simulink model "Q2_Model"  (R2016b)
settings: Solver=VariableStepAuto  StartTime=0.0  StopTime=100  RelTol=1e-10  AbsTol=1e-10
values from neighbouring files (symbols this model uses):
  c_a = 0.1    [CSD_HW_1_Script.m]
  D_v = 1e-2    (= 0.01)    [CSD_HW_1_Script.m]
  ddx_height = 5    [CSD_HW_1_Script.m]
  ddx_width = 30/ddx_height    (= 6)    [CSD_HW_1_Script.m]
  gear = 2    [CSD_HW_1_Script.m]
  J = 0.07    [CSD_HW_1_Script.m]
  K_t = 0.46    [CSD_HW_1_Script.m]
  l = 0.3    [CSD_HW_1_Script.m]
  m = 0.8    [CSD_HW_1_Script.m]
  N = 3    [CSD_HW_1_Script.m]    (also in Plotshit.m)
  R = 0.1    [CSD_HW_1_Script.m]    (also in Plotshit.m)
  Step_Height = 0    [CSD_HW_1_Script.m]
  T_sl = 2    [CSD_HW_1_Script.m]
  T_st = 2.6    [CSD_HW_1_Script.m]
  V_max = 20    [CSD_HW_1_Script.m]
undefined symbols (not defined in the file or in its folder): magnitude
libraries: cstblocks x1
settings Model: Creator=nadav  LastModifiedBy=nadav

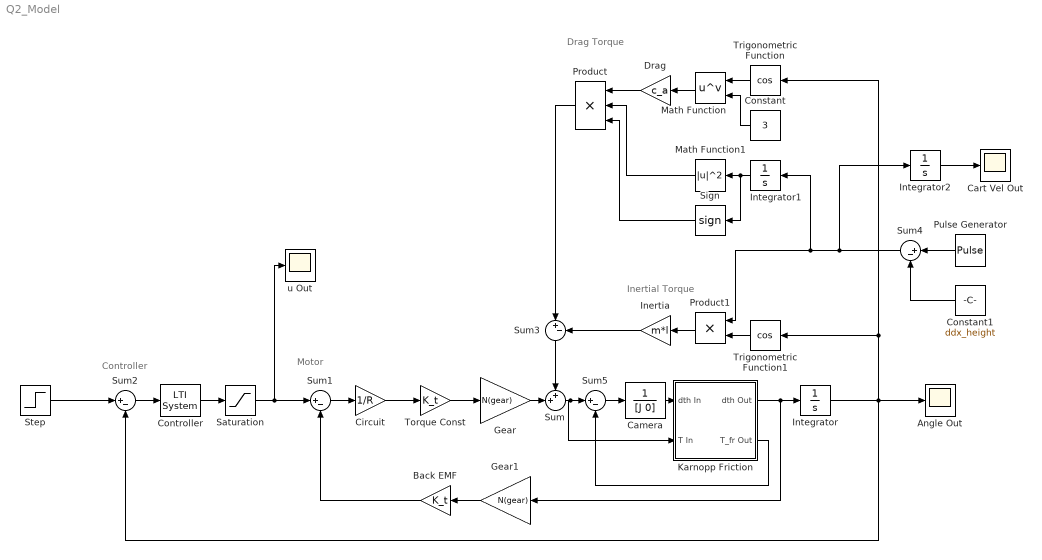
== system Q2_Model ==
  note: Inertial Torque
  note: Drag Torque
  note: Controller
  note: Motor
  Angle Out : Scope
  Back EMF : Gain  Gain=K_t
  Camera : TransferFcn  Denominator=[J 0]
  Cart Vel Out : Scope
  Circuit : Gain  Gain=1/R
  Constant : Constant  Value=3
  Constant1 : Constant  Value=ddx_height
  Controller : cstblocks/LTI System  sys=C  IC=[]
  Drag : Gain  Gain=c_a
  Gear : Gain  Gain=N(gear)
  Gear1 : Gain  Gain=N(gear)
  Inertia : Gain  Gain=m*l
  Integrator : Integrator
  Integrator1 : Integrator
  Integrator2 : Integrator
  Karnopp Friction : Subsystem
  Math Function : Math  Operator=pow  SaturateOnIntegerOverflow=on
  Math Function1 : Math  Operator=magnitude^2  SaturateOnIntegerOverflow=on
  Product : Product  Inputs=3
  Product1 : Product
  Pulse Generator : DiscretePulseGenerator  PulseType=Time based  Amplitude=2*ddx_height  Period=4*ddx_width  PulseWidth=50  PhaseDelay=-ddx_width
  Saturation : Saturate  UpperLimit=V_max  LowerLimit=-V_max
  Sign : Signum
  Step : Step  Time=0  After=Step_Height  SampleTime=0
  Sum : Sum  Inputs=++|
  Sum{1..5} (5 alike) : Sum  Inputs=|+-
  Torque Const : Gain  Gain=K_t
  Trigonometric Function : Trigonometry  Operator=cos
  Trigonometric Function1 : Trigonometry  Operator=cos
  u Out : Scope
  wires:
  Karnopp Friction/1(dth Out) -> Gear1/1, Integrator/1
  Camera/1 -> Karnopp Friction/1(dth In)
  Gear/1 -> Sum/2
  Torque Const/1 -> Gear/1
  Circuit/1 -> Torque Const/1
  Gear1/1 -> Back EMF/1
  Back EMF/1 -> Sum1/2
  Sum1/1 -> Circuit/1
  Sum2/1 -> Controller/1
  Integrator/1 -> Sum2/2, Trigonometric Function/1, Trigonometric Function1/1, Angle Out/1
  Saturation/1 -> u Out/1, Sum1/1
  Controller/1 -> Saturation/1
  Step/1 -> Sum2/1
  Sum4/1 -> Integrator2/1, Product1/1, Integrator1/1
  Trigonometric Function/1 -> Math Function/1
  Constant/1 -> Math Function/2
  Math Function/1 -> Drag/1
  Integrator1/1 -> Sign/1, Math Function1/1
  Sum3/1 -> Sum/1
  Drag/1 -> Product/1
  Math Function1/1 -> Product/2
  Product/1 -> Sum3/1
  Trigonometric Function1/1 -> Product1/2
  Product1/1 -> Inertia/1
  Inertia/1 -> Sum3/2
  Sign/1 -> Product/3
  Pulse Generator/1 -> Sum4/1
  Constant1/1 -> Sum4/2
  Integrator2/1 -> Cart Vel Out/1
  Sum/1 -> Karnopp Friction/2(T In), Sum5/1
  Sum5/1 -> Camera/1
  Karnopp Friction/2(T_fr Out) -> Sum5/2

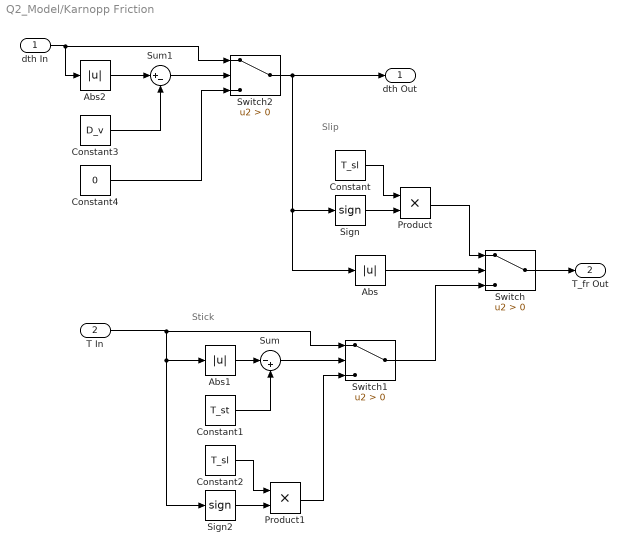
== system Q2_Model/Karnopp Friction ==
  note: Stick
  note: Slip
  dth In : Inport
  T In : Inport  Port=2
  Abs : Abs
  Abs1 : Abs
  Abs2 : Abs
  Constant : Constant  Value=T_sl
  Constant1 : Constant  Value=T_st
  Constant2 : Constant  Value=T_sl
  Constant3 : Constant  Value=D_v
  Constant4 : Constant  Value=0
  Product : Product
  Product1 : Product
  Sign : Signum
  Sign2 : Signum
  Sum : Sum  Inputs=|-+
  Sum1 : Sum  Inputs=|+-
  Switch : Switch  Criteria=u2 > Threshold
  Switch1 : Switch  Criteria=u2 > Threshold
  Switch2 : Switch  Criteria=u2 > Threshold
  dth Out : Outport
  T_fr Out : Outport  Port=2
  wires:
  Product/1 -> Switch/1
  Sum/1 -> Switch1/2
  Constant1/1 -> Sum/2
  Abs1/1 -> Sum/1
  Constant/1 -> Product/1
  Sign/1 -> Product/2
  T In/1 -> Sign2/1, Abs1/1, Switch1/1
  Sign2/1 -> Product1/2
  Product1/1 -> Switch1/3
  Abs/1 -> Switch/2
  dth In/1 -> Abs2/1, Switch2/1
  Constant2/1 -> Product1/1
  Switch1/1 -> Switch/3
  Switch2/1 -> dth Out/1, Abs/1, Sign/1
  Switch/1 -> T_fr Out/1
  Constant3/1 -> Sum1/2
  Abs2/1 -> Sum1/1
  Sum1/1 -> Switch2/2
  Constant4/1 -> Switch2/3
